simulink model "CVSG"  (R2024b)
settings: Solver=ode4  StartTime=0.0  StopTime=60  FixedStep=1e-5  RelTol=1e-3
values from neighbouring files (symbols this model uses):
  Dp = 2.087054162363824e+03    (= 2087.05416236)    [CVSGm.m]
  Dq = 0.686969675951841    (= 0.686969675952)    [CVSGm.m]
  Kp = 0.007666307989764    (= 0.00766630798976)    [CVSGm.m]
  Kq = 0.115300461672244    (= 0.115300461672)    [CVSGm.m]
undefined symbols (not defined in the file or in its folder): Filter, Ls, params
libraries: spsCurrentMeasurementLib x6, spsParallelRLCBranchLib x6, spsIGBTDiodeLib x6, spsSeriesRLCBranchLib x6, simulink x4, spsVoltageMeasurementLib x4, spsVariableInductorLib x3, spsVariableResistorLib x3, spsMeanLib x2, spsDCVoltageSourceLib x1, spsThreePhaseSourceLib x1, spsThreePhaseVIMeasurementLib x1
settings Model: SimulationMode=accelerator  Creator=Admin  LastModifiedBy=ACER
settings DataIOCC: SaveOutput=off  DSMLogging=off  SaveTime=off  ReturnWorkspaceOutputs=off
settings OptimizationCC: EfficientMapNaN2IntZero=off  AccelVerboseBuild=on
settings DebuggingCC: SignalInfNanChecking=error  CheckMatrixSingularityMsg=error  UnconnectedInputMsg=warning  UnconnectedOutputMsg=warning  UnconnectedLineMsg=warning
settings HardwareCC: TargetBitPerPointer=64  TargetBitPerSizeT=64  TargetBitPerPtrDiffT=64  TargetLongLongMode=on  TargetIntDivRoundTo=Zero  TargetEndianess=LittleEndian  TargetWordSize=64  TargetHWDeviceType=MATLAB Host  ProdEqTarget=off
settings ModelReferenceCC: EnableRefExpFcnMdlSchedulingChecks=on
settings SFSimCC: CustomCodeUndefinedFunction=UseInterfaceOnly
settings RTWCC: GPUComputeCapability=3.5
settings CodeAppCC: MaxIdLength=128
settings GRTTargetCC: TargetLangStandard=C89/C90 (ANSI)  CombineOutputUpdateFcns=off  GRTInterface=on

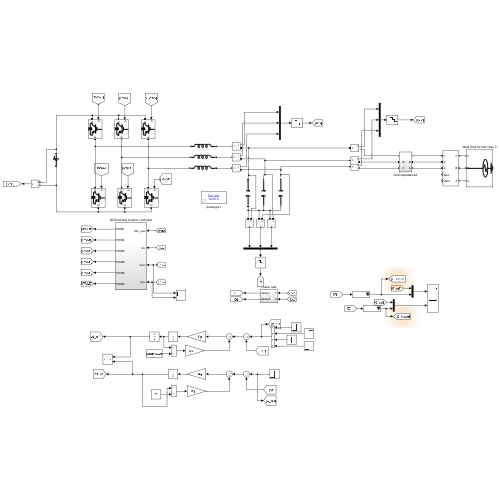
[thumbnail: Simulink's stored preview of the top-level diagram]
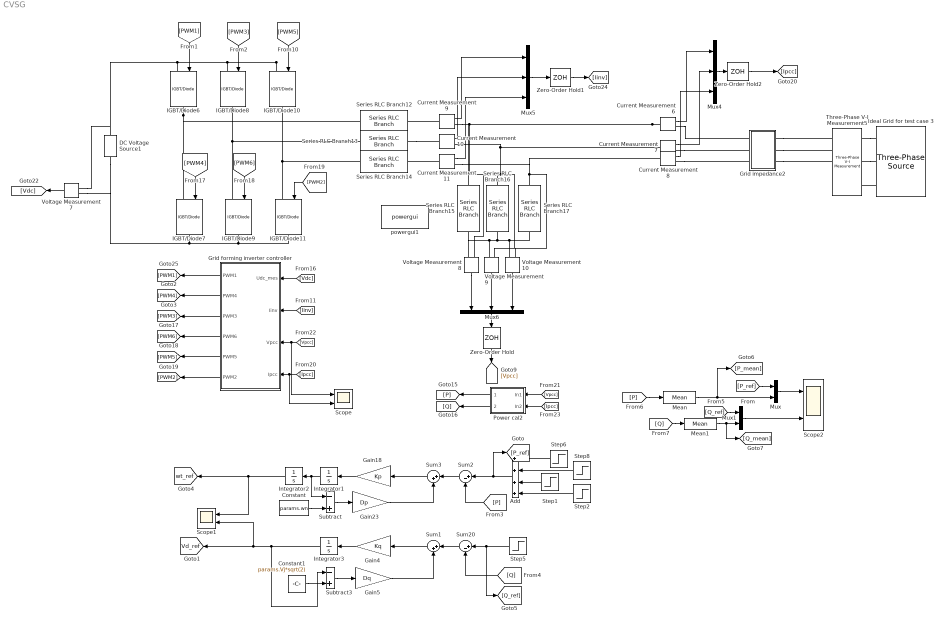
== system CVSG ==
  Add : Sum  Inputs=++++
  Constant : Constant  Value=params.wn
  Constant1 : Constant  Value=params.Vj*sqrt(2)
  Current Measurement{6..11} (6 alike) : spsCurrentMeasurementLib/Current Measurement  PhasorSimulation=off  OutputType=Complex  PSBequivalent=0
  DC Voltage Source1 : spsDCVoltageSourceLib/DC Voltage Source  Amplitude=params.Vdc  Measurements=None
  Gain18 : Gain  Gain=Kp
  Gain23 : Gain  Gain=Dp
  Gain4 : Gain  Gain=Kq
  Gain5 : Gain  Gain=Dq
  Grid forming inverter controller : Subsystem
  Grid impedance2 : Subsystem
  IGBT/Diode{6..11} (6 alike) : spsIGBTDiodeLib/IGBT//Diode  Ron=1e-3  Rs=1e5  Cs=inf  Measurements=off
  Ideal Grid for test case 3 : spsThreePhaseSourceLib/Three-Phase Source  InternalConnection=Yg  VoltagePhases=off  Voltage=params.Vj*sqrt(3)  PhaseAngle=0  Voltage_phases=[25e3 25e3 25e3]/sqrt(3)  PhaseAngles_phases=[0 -120 +120]  Frequency=params.f0  NonIdealSource=off  SpecifyImpedance=on  Resistance=0.8929  Inductance=16.58e-3  ShortCircuitLevel=params.SCR*params.S_rated  BaseVoltage=params.Vll_rms  XRratio=params.XR  BusType=swing  Pref=1e3  Qref=0  Prefabc=[10e3, 10e3, 10e3]  Qrefabc=[0, 0, 0]  Qmin=-inf  Qmax=inf
  Integrator1 : Integrator
  Integrator2 : Integrator
  Integrator3 : Integrator
  Mean : spsMeanLib/Mean  Freq=60  Vinit=0  Ts=0
  Mean1 : spsMeanLib/Mean  Freq=60  Vinit=0  Ts=0
  Mux : Mux  Inputs=2
  Mux1 : Mux  Inputs=2
  Mux4 : Mux  Inputs=3
  Mux5 : Mux  Inputs=3
  Mux6 : Mux  Inputs=3
  Power cal2 : Subsystem
  Scope : Scope  NumInputPorts=2
  Scope1 : Scope  NumInputPorts=2
  Scope2 : Scope  NumInputPorts=2
  Series RLC Branch12 : spsSeriesRLCBranchLib/Series RLC Branch  LConnTagsString=__new0  RConnTagsString=__new0  BranchType=L  Resistance=Filter.Rs_1  Inductance=params.Filter.Ls_1  SetiL0=off  InitialCurrent=1  Capacitance=1e-6  Setx0=off  InitialVoltage=0  Measurements=None
  Series RLC Branch13 : spsSeriesRLCBranchLib/Series RLC Branch  LConnTagsString=__new0  RConnTagsString=__new0  BranchType=L  Resistance=Filter.Rs_1  Inductance=params.Filter.Ls_1  SetiL0=off  InitialCurrent=1  Capacitance=1e-6  Setx0=off  InitialVoltage=0  Measurements=None
  Series RLC Branch14 : spsSeriesRLCBranchLib/Series RLC Branch  LConnTagsString=__new0  RConnTagsString=__new0  BranchType=L  Resistance=Filter.Rs_1  Inductance=params.Filter.Ls_1  SetiL0=off  InitialCurrent=1  Capacitance=1e-6  Setx0=off  InitialVoltage=0  Measurements=None
  Series RLC Branch15 : spsSeriesRLCBranchLib/Series RLC Branch  LConnTagsString=__new0  RConnTagsString=__new0  BranchType=C  Resistance=1  Inductance=Ls  SetiL0=off  InitialCurrent=0  Capacitance=params.Filter.Cs  Setx0=off  InitialVoltage=0  Measurements=None
  Series RLC Branch16 : spsSeriesRLCBranchLib/Series RLC Branch  LConnTagsString=__new0  RConnTagsString=__new0  BranchType=C  Resistance=1  Inductance=Ls  SetiL0=off  InitialCurrent=0  Capacitance=params.Filter.Cs  Setx0=off  InitialVoltage=0  Measurements=None
  Series RLC Branch17 : spsSeriesRLCBranchLib/Series RLC Branch  LConnTagsString=__new0  RConnTagsString=__new0  BranchType=C  Resistance=1  Inductance=Ls  SetiL0=off  InitialCurrent=0  Capacitance=params.Filter.Cs  Setx0=off  InitialVoltage=0  Measurements=None
  Step1 : Step  Time=70  After=0.5e3  SampleTime=0
  Step2 : Step  Time=70  After=0.5e3  SampleTime=0
  Step5 : Step  Time=50  Before=1e3  After=1.5e3  SampleTime=0
  Step6 : Step  Time=10  Before=2e3  After=2.5e3  SampleTime=0
  Step8 : Step  Time=30  After=0.5e3  SampleTime=0
  Subtract : Sum  Inputs=-+
  Subtract3 : Sum  Inputs=-+
  Sum1 : Sum  Inputs=|++
  Sum2 : Sum  Inputs=|+-
  Sum20 : Sum  Inputs=|+-
  Sum3 : Sum  Inputs=|++
  Three-Phase V-I Measurement5 : spsThreePhaseVIMeasurementLib/Three-Phase V-I Measurement  VoltageMeasurement=phase-to-ground  SetLabelV=off  LabelV=Vabc  Vpu=off  VpuLL=off  CurrentMeasurement=yes  SetLabelI=off  LabelI=Iabc  Ipu=off  Pbase=100e6  Vbase=500e3  OutputType=Complex  PhasorSimulation=off  PSBequivalent=0
  Voltage Measurement{7..10} (4 alike) : spsVoltageMeasurementLib/Voltage Measurement  PhasorSimulation=off  OutputType=Complex  PSBequivalent=0
  Zero-Order Hold : ZeroOrderHold  SampleTime=5e-5
  Zero-Order Hold1 : ZeroOrderHold  SampleTime=5e-5
  Zero-Order Hold2 : ZeroOrderHold  SampleTime=5e-5
  powergui1 : sps_lib/powergui  Priority=1  SimulationMode=Discrete  SampleTime=1e-5  frequency=60  Iterations=50  frequencyindice=0  Pbase=100e6  ErrMax=1e-4  UnitsV=kV  UnitsW=MW  buscounter=0  FunctionMessages=off  echomessages=off  EnableUseOfTLC=off  CurrentSourceSwitches=off  DisableSnubberDevices=off  DisableRonSwitches=off  DisableVfSwitches=off  DisplayEquations=off  AutomaticDiscreteSolvers=on  SolverType=Tustin/Backward Euler (TBE)  Interpol=off  ExternalGateDelay=off  methode=off  Ts=100  x0status=blocks  SPID=on  SwTol=0  HookPort=off  NonlinearTolerance=0  nMaxIteration=15  ContinueOnMaxIteration=off  RestoreLinks=warning  ResistiveCurrentMeasurement=off  Frange=[0:2:500]  Ylog=off  Xlog=on  ShowGrid=off  save=off  variable=ZData  structure=0  ZoomFFT=off  StartTime=0.0  cycles=1  DisplayStyle=1  fundamental=60  FreqAxis=off  MaxFrequency=1000  frequencyindicesteady=1  RmsSteady=1  display=off
  tag scope: Vd_ref=global, wt_ref=global
  wires:
  [Iinv] -> Grid forming inverter controller/2(Iinv)
  Grid forming inverter controller/1(PWM1) -> [PWM1]
  Grid forming inverter controller/4("PWM6 ") -> [PWM6]
  Grid forming inverter controller/6(PWM2) -> [PWM2]
  Voltage Measurement7/1 -> [Vdc]
  Grid forming inverter controller/5(PWM5) -> [PWM5]
  Voltage Measurement9/1 -> Mux6/2
  Mux5/1 -> Zero-Order Hold1/1
  [PWM6] -> IGBT/Diode9/1
  [PWM1] -> IGBT/Diode6/1
  [Ipcc] -> Scope/2, Grid forming inverter controller/4(Ipcc)
  [Vdc] -> Grid forming inverter controller/1(Udc_mes)
  [Vpcc] -> Scope/1, Grid forming inverter controller/3(Vpcc)
  Grid forming inverter controller/3(PWM3) -> [PWM3]
  Grid forming inverter controller/2("PWM4 ") -> [PWM4]
  Current Measurement11/1 -> Mux5/3
  Voltage Measurement10/1 -> Mux6/3
  [PWM2] -> IGBT/Diode11/1
  Mux4/1 -> Zero-Order Hold2/1
  [PWM4] -> IGBT/Diode7/1
  Mux6/1 -> Zero-Order Hold/1
  [PWM5] -> IGBT/Diode10/1
  Current Measurement8/1 -> Mux4/3
  Voltage Measurement8/1 -> Mux6/1
  Current Measurement9/1 -> Mux5/1
  Current Measurement7/1 -> Mux4/2
  Current Measurement6/1 -> Mux4/1
  Current Measurement10/1 -> Mux5/2
  [PWM3] -> IGBT/Diode8/1
  Power cal2/2(deltay2) -> [Q]
  Power cal2/1(deltay1) -> [P]
  [Vpcc] -> Power cal2/1(In1)
  [Ipcc] -> Power cal2/2(In2)
  Zero-Order Hold/1 -> [Vpcc]
  Zero-Order Hold1/1 -> [Iinv]
  Zero-Order Hold2/1 -> [Ipcc]
  Step8/1 -> Add/2
  Constant/1 -> Subtract/2
  Gain18/1 -> Integrator1/1
  Sum1/1 -> Gain4/1
  Gain5/1 -> Sum1/2
  Sum3/1 -> Gain18/1
  [Q] -> Sum20/2
  Integrator1/1 -> Subtract/1, Integrator2/1
  Constant1/1 -> Subtract3/2
  [P] -> Sum2/2
  Sum2/1 -> Sum3/1
  Integrator3/1 -> Scope1/2, [Vd_ref], Subtract3/1
  Sum20/1 -> Sum1/1
  Integrator2/1 -> [wt_ref], Scope1/1
  Subtract/1 -> Gain23/1
  Gain4/1 -> Integrator3/1
  Gain23/1 -> Sum3/2
  Subtract3/1 -> Gain5/1
  Mux/1 -> Scope2/1
  Mux1/1 -> Scope2/2
  Mean/1 -> [P_mean], Mux/2
  [P_ref] -> Mux/1
  [Q_ref] -> Mux1/1
  [P] -> Mean/1
  [Q] -> Mean1/1
  Step6/1 -> Add/1
  Add/1 -> [P_ref], Sum2/1
  Step1/1 -> Add/3
  Step2/1 -> Add/4
  Step5/1 -> [Q_ref], Sum20/1
  Mean1/1 -> [Q_mean], Mux1/2
  connections:
  Series RLC Branch14/LConn1 -- IGBT/Diode10/RConn1 -- IGBT/Diode11/LConn1
  Series RLC Branch17/LConn1 -- Current Measurement11/RConn1 -- Current Measurement8/LConn1 -- Voltage Measurement10/LConn1
  IGBT/Diode6/RConn1 -- Series RLC Branch12/LConn1 -- IGBT/Diode7/LConn1
  Voltage Measurement10/LConn2 -- Series RLC Branch17/RConn1 -- Voltage Measurement8/LConn2 -- Series RLC Branch15/RConn1 -- Voltage Measurement9/LConn2 -- Series RLC Branch16/RConn1
  Current Measurement6/LConn1 -- Series RLC Branch15/LConn1 -- Voltage Measurement8/LConn1 -- Current Measurement9/RConn1
  IGBT/Diode10/LConn1 -- DC Voltage Source1/RConn1 -- Voltage Measurement7/LConn1 -- IGBT/Diode6/LConn1 -- IGBT/Diode8/LConn1
  IGBT/Diode7/RConn1 -- IGBT/Diode11/RConn1 -- IGBT/Diode9/RConn1 -- Voltage Measurement7/LConn2 -- DC Voltage Source1/LConn1
  Series RLC Branch13/LConn1 -- IGBT/Diode8/RConn1 -- IGBT/Diode9/LConn1
  Current Measurement7/LConn1 -- Current Measurement10/RConn1 -- Series RLC Branch16/LConn1 -- Voltage Measurement9/LConn1
  Current Measurement7/RConn1 -- Grid impedance2/LConn2
  Current Measurement11/LConn1 -- Series RLC Branch14/RConn1
  Current Measurement8/RConn1 -- Grid impedance2/LConn3
  Series RLC Branch13/RConn1 -- Current Measurement10/LConn1
  Current Measurement9/LConn1 -- Series RLC Branch12/RConn1
  Current Measurement6/RConn1 -- Grid impedance2/LConn1
  Grid impedance2/RConn1 -- Three-Phase V-I Measurement5/RConn3
  Three-Phase V-I Measurement5/LConn2 -- Ideal Grid for test case 3/RConn2
  Three-Phase V-I Measurement5/LConn3 -- Ideal Grid for test case 3/RConn3
  Grid impedance2/RConn2 -- Three-Phase V-I Measurement5/RConn2
  Ideal Grid for test case 3/RConn1 -- Three-Phase V-I Measurement5/LConn1
  Grid impedance2/RConn3 -- Three-Phase V-I Measurement5/RConn1

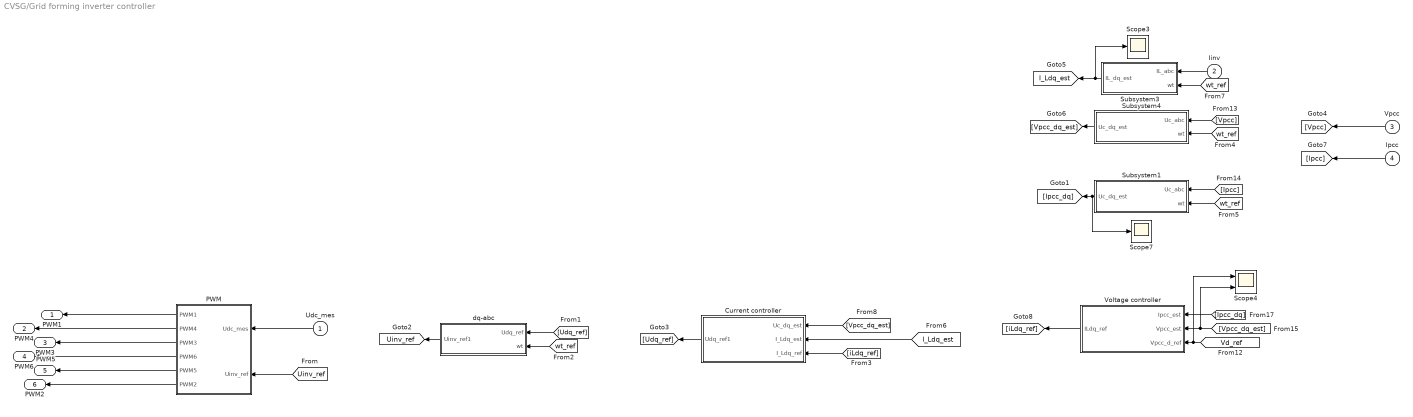
== system CVSG/Grid forming inverter controller ==
  Udc_mes : Inport
  Iinv : Inport  Port=2
  Vpcc : Inport  Port=3
  Ipcc : Inport  Port=4
  Current controller : Subsystem
  PWM : Subsystem
  Scope3 : Scope
  Scope4 : Scope  NumInputPorts=2
  Scope7 : Scope
  Subsystem1 : Subsystem
  Subsystem3 : Subsystem
  Subsystem4 : Subsystem
  Voltage controller : Subsystem
  dq-abc : Subsystem
  PWM1 : Outport
  "PWM4 " : Outport  Port=2
  PWM3 : Outport  Port=3
  "PWM6 " : Outport  Port=4
  PWM5 : Outport  Port=5
  PWM2 : Outport  Port=6
  tag scope: I_Ldq_est=global, Uinv_ref=global
  wires:
  [Vpcc_dq_est] -> Current controller/1(Uc_dq_est)
  PWM/4("PWM6 ") -> "PWM6 "/1
  Udc_mes/1 -> PWM/1(Udc_mes)
  [I_Ldq_est] -> Current controller/2(I_Ldq_est)
  Subsystem4/1(Uc_dq_est) -> [Vpcc_dq_est]
  Current controller/1(Udq_ref1) -> [Udq_ref]
  [wt_ref] -> Subsystem3/2(wt)
  dq-abc/1(Uinv_ref1) -> [Uinv_ref]
  [wt_ref] -> dq-abc/2(wt)
  Iinv/1 -> Subsystem3/1(IL_abc)
  PWM/3(PWM3) -> PWM3/1
  Subsystem3/1(IL_dq_est) -> Scope3/1, [I_Ldq_est]
  [wt_ref] -> Subsystem4/2(wt)
  PWM/1(PWM1) -> PWM1/1
  PWM/5(PWM5) -> PWM5/1
  PWM/6(PWM2) -> PWM2/1
  PWM/2("PWM4 ") -> "PWM4 "/1
  [Udq_ref] -> dq-abc/1(Udq_ref)
  [Uinv_ref] -> PWM/2(Uinv_ref)
  [Ipcc_dq] -> Voltage controller/1(Ipcc_est)
  Voltage controller/1(ILdq_ref) -> [iLdq_ref]
  [Vpcc_dq_est] -> Scope4/2, Voltage controller/2(Vpcc_est)
  [iLdq_ref] -> Current controller/3(I_Ldq_ref)
  [wt_ref] -> Subsystem1/2(wt)
  Subsystem1/1(Uc_dq_est) -> [Ipcc_dq], Scope7/1
  Vpcc/1 -> [Vpcc]
  Ipcc/1 -> [Ipcc]
  [Vpcc] -> Subsystem4/1(Uc_abc)
  [Ipcc] -> Subsystem1/1(Uc_abc)
  [Vd_ref] -> Scope4/1, Voltage controller/3(Vpcc_d_ref)

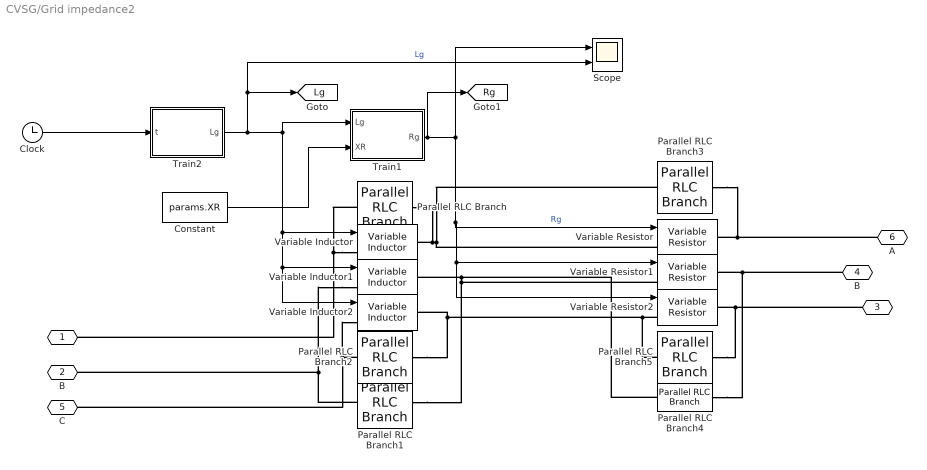
== system CVSG/Grid impedance2 ==
  Clock : Clock
      settings: Decimation=150
  Constant : Constant  Value=params.XR
  Parallel RLC Branch{,1..5} (6 alike) : spsParallelRLCBranchLib/Parallel RLC Branch  LConnTagsString=a  RConnTagsString=__new0  BranchType=R  Resistance=1e6  Inductance=1e-3  SetiL0=off  InitialCurrent=0  Capacitance=1e-6  Setx0=off  InitialVoltage=0  Measurements=None
  Scope : Scope  NumInputPorts=2
  Train1 : MATLAB Function  TreatAsAtomicUnit=on
  Train2 : MATLAB Function  TreatAsAtomicUnit=on
  Variable Inductor : spsVariableInductorLib/Variable Inductor  methode=Backward Euler  Labsmin=1e-6  Initialize=off  iL0=0  L0=1e-3  Vl0=-0.0024759
  Variable Inductor1 : spsVariableInductorLib/Variable Inductor  methode=Backward Euler  Labsmin=1e-6  Initialize=off  iL0=0  L0=1e-3  Vl0=67.3622
  Variable Inductor2 : spsVariableInductorLib/Variable Inductor  methode=Backward Euler  Labsmin=1e-6  Initialize=off  iL0=0  L0=1e-3  Vl0=-67.3597
  Variable Resistor : spsVariableResistorLib/Variable Resistor  Rabsmin=1e-3
  Variable Resistor1 : spsVariableResistorLib/Variable Resistor  Rabsmin=1e-3
  Variable Resistor2 : spsVariableResistorLib/Variable Resistor  Rabsmin=1e-3
  "   " : PMIOPort  Side=Left
  "   B" : PMIOPort  Port=2  Side=Left
  "  " : PMIOPort  Port=3  Side=Right
  "  B" : PMIOPort  Port=4  Side=Right
  "   C" : PMIOPort  Port=5  Side=Left
  "  A" : PMIOPort  Port=6  Side=Right
  tag scope: Lg=global, Rg=global
  wires:
  Train1/1(Rg) -> [Rg], Scope/1, Variable Resistor/1, Variable Resistor1/1, Variable Resistor2/1  "Rg"
  Clock/1 -> Train2/1(t)
  Train2/1(Lg) -> [Lg], Scope/2, Variable Inductor/1, Variable Inductor1/1, Variable Inductor2/1, Train1/1(Lg)  "Lg"
  Constant/1 -> Train1/2(XR)
  connections:
  Variable Resistor1/LConn1 -- Variable Inductor1/RConn1 -- Parallel RLC Branch4/LConn1 -- Parallel RLC Branch1/RConn1
  Variable Resistor2/LConn1 -- Parallel RLC Branch5/LConn1 -- Variable Inductor2/RConn1 -- Parallel RLC Branch2/RConn1
  Variable Resistor1/RConn1 -- Parallel RLC Branch4/RConn1 -- "  B"/RConn1
  Variable Resistor2/RConn1 -- Parallel RLC Branch5/RConn1 -- "  "/RConn1
  Variable Resistor/RConn1 -- Parallel RLC Branch3/RConn1 -- "  A"/RConn1
  Variable Inductor/LConn1 -- "   "/RConn1 -- Parallel RLC Branch/LConn1
  Variable Inductor/RConn1 -- Parallel RLC Branch3/LConn1 -- Variable Resistor/LConn1 -- Parallel RLC Branch/RConn1
  Variable Inductor1/LConn1 -- "   B"/RConn1 -- Parallel RLC Branch1/LConn1
  Variable Inductor2/LConn1 -- "   C"/RConn1 -- Parallel RLC Branch2/LConn1

== system CVSG/Power cal2 ==
  In1 : Inport
  In2 : Inport  Port=2
  Demux10 : Demux  Outputs=3
  Demux11 : Demux  Outputs=3
  Subsystem8 : Subsystem
  Subsystem9 : Subsystem
  p3 : Subsystem
  q3 : Subsystem
  deltay1 : Outport
  deltay2 : Outport  Port=2
  wires:
  In1/1 -> Demux11/1
  In2/1 -> Demux10/1
  q3/1(deltay2) -> deltay2/1
  Demux10/1 -> Subsystem8/1(xa)
  Demux11/2 -> Subsystem9/2(xb)
  Demux11/1 -> Subsystem9/1(xa)
  Subsystem9/2(xbeta) -> q3/2(Beta), p3/2(Beta)
  p3/1(deltay1) -> deltay1/1
  Demux10/3 -> Subsystem8/3(xc)
  Subsystem9/1(xalpha) -> q3/1(Alpha), p3/1(Alpha)
  Demux10/2 -> Subsystem8/2(xb)
  Subsystem8/2(xbeta) -> q3/4(xbeta), p3/4(xbeta)
  Demux11/3 -> Subsystem9/3(xc)
  Subsystem8/1(xalpha) -> q3/3(xalpha), p3/3(xalpha)

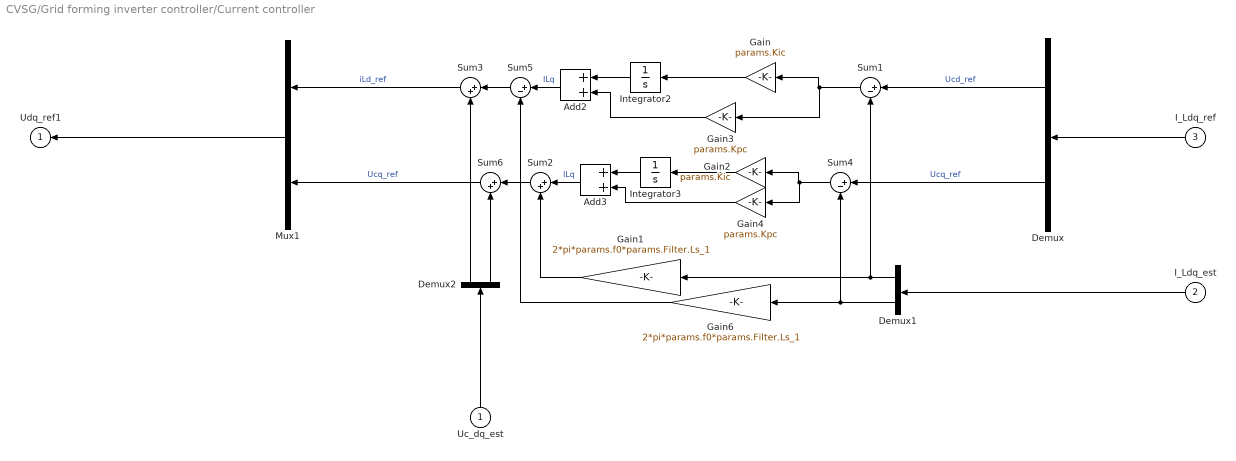
== system CVSG/Grid forming inverter controller/Current controller ==
  Uc_dq_est : Inport
  I_Ldq_est : Inport  Port=2
  I_Ldq_ref : Inport  Port=3
  Add2 : Sum
  Add3 : Sum
  Demux : Demux  Outputs=2
  Demux1 : Demux  Outputs=2
  Demux2 : Demux  Outputs=2
  Gain : Gain  Gain=params.Kic
  Gain1 : Gain  Gain=2*pi*params.f0*params.Filter.Ls_1
  Gain2 : Gain  Gain=params.Kic
  Gain3 : Gain  Gain=params.Kpc
  Gain4 : Gain  Gain=params.Kpc
  Gain6 : Gain  Gain=2*pi*params.f0*params.Filter.Ls_1
  Integrator2 : Integrator
  Integrator3 : Integrator
  Mux1 : Mux  Inputs=2
  Sum1 : Sum  Inputs=|+-
  Sum2 : Sum  Inputs=|++
  Sum3 : Sum  Inputs=|++
  Sum4 : Sum  Inputs=|+-
  Sum5 : Sum  Inputs=|+-
  Sum6 : Sum  Inputs=|++
  Udq_ref1 : Outport  InitialOutput=0  VectorParamsAs1DForOutWhenUnconnected=off
  wires:
  I_Ldq_ref/1 -> Demux/1
  Demux2/2 -> Sum6/2
  Sum2/1 -> Sum6/1
  I_Ldq_est/1 -> Demux1/1
  Sum3/1 -> Mux1/1  "iLd_ref"
  Demux/2 -> Sum4/1  "Ucq_ref"
  Gain1/1 -> Sum2/2
  Sum6/1 -> Mux1/2  "Ucq_ref"
  Demux2/1 -> Sum3/2
  Sum5/1 -> Sum3/1
  Mux1/1 -> Udq_ref1/1
  Gain6/1 -> Sum5/2
  Uc_dq_est/1 -> Demux2/1
  Demux1/2 -> Gain6/1, Sum4/2
  Demux/1 -> Sum1/1  "Ucd_ref"
  Demux1/1 -> Sum1/2, Gain1/1
  Add2/1 -> Sum5/1  "ILq"
  Add3/1 -> Sum2/1  "ILq"
  Integrator2/1 -> Add2/1
  Integrator3/1 -> Add3/1
  Gain/1 -> Integrator2/1
  Sum1/1 -> Gain3/1, Gain/1
  Gain2/1 -> Integrator3/1
  Sum4/1 -> Gain4/1, Gain2/1
  Gain3/1 -> Add2/2
  Gain4/1 -> Add3/2

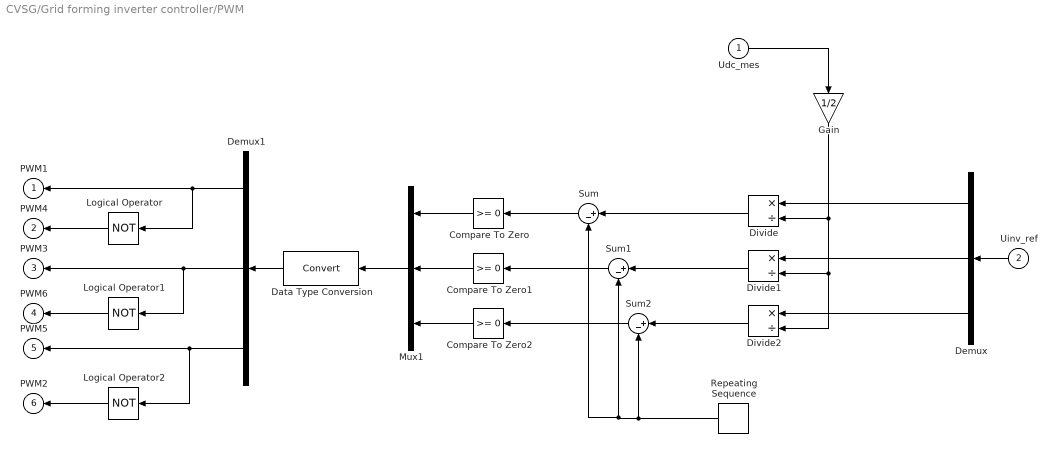
== system CVSG/Grid forming inverter controller/PWM ==
  Udc_mes : Inport
  Uinv_ref : Inport  Port=2
  Compare To Zero : simulink/Logic and Bit Operations/Compare To Zero  relop=>=  OutDataTypeStr=boolean
  Compare To Zero1 : simulink/Logic and Bit Operations/Compare To Zero  relop=>=  OutDataTypeStr=boolean
  Compare To Zero2 : simulink/Logic and Bit Operations/Compare To Zero  relop=>=  OutDataTypeStr=boolean
  Data Type Conversion : DataTypeConversion  SaturateOnIntegerOverflow=off  RndMeth=Floor
  Demux : Demux  Outputs=3
  Demux1 : Demux  Outputs=3
  Divide : Product  Inputs=*/
  Divide1 : Product  Inputs=*/
  Divide2 : Product  Inputs=*/
  Gain : Gain  Gain=1/2
  Logical Operator : Logic  Operator=NOT  AllPortsSameDT=off  OutDataTypeStr=boolean
  Logical Operator1 : Logic  Operator=NOT  AllPortsSameDT=off  OutDataTypeStr=boolean
  Logical Operator2 : Logic  Operator=NOT  AllPortsSameDT=off  OutDataTypeStr=boolean
  Mux1 : Mux  Inputs=3
  Repeating Sequence : simulink/Sources/Repeating Sequence  rep_seq_t=[0 params.Ts/2 params.Ts]  rep_seq_y=[-1 1 -1]
  Sum : Sum  Inputs=|+-
  Sum1 : Sum  Inputs=|+-
  Sum2 : Sum  Inputs=|+-
  PWM1 : Outport  InitialOutput=0  VectorParamsAs1DForOutWhenUnconnected=off
  "PWM4 " : Outport  Port=2  InitialOutput=0  VectorParamsAs1DForOutWhenUnconnected=off
  PWM3 : Outport  Port=3  InitialOutput=0  VectorParamsAs1DForOutWhenUnconnected=off
  "PWM6 " : Outport  Port=4  InitialOutput=0  VectorParamsAs1DForOutWhenUnconnected=off
  PWM5 : Outport  Port=5  InitialOutput=0  VectorParamsAs1DForOutWhenUnconnected=off
  PWM2 : Outport  Port=6  InitialOutput=0  VectorParamsAs1DForOutWhenUnconnected=off
  wires:
  Repeating Sequence/1 -> Sum/2, Sum1/2, Sum2/2
  Sum1/1 -> Compare To Zero1/1
  Mux1/1 -> Data Type Conversion/1
  Divide2/1 -> Sum2/1
  Divide/1 -> Sum/1
  Logical Operator/1 -> "PWM4 "/1
  Sum2/1 -> Compare To Zero2/1
  Divide1/1 -> Sum1/1
  Demux/1 -> Divide/1
  Uinv_ref/1 -> Demux/1
  Demux1/2 -> PWM3/1, Logical Operator1/1
  Demux1/3 -> PWM5/1, Logical Operator2/1
  Compare To Zero2/1 -> Mux1/3
  Compare To Zero1/1 -> Mux1/2
  Demux/2 -> Divide1/1
  Logical Operator2/1 -> PWM2/1
  Logical Operator1/1 -> "PWM6 "/1
  Udc_mes/1 -> Gain/1
  Demux/3 -> Divide2/1
  Sum/1 -> Compare To Zero/1
  Gain/1 -> Divide/2, Divide1/2, Divide2/2
  Demux1/1 -> PWM1/1, Logical Operator/1
  Data Type Conversion/1 -> Demux1/1
  Compare To Zero/1 -> Mux1/1

== system CVSG/Grid forming inverter controller/Subsystem1 ==
  Uc_abc : Inport
  wt : Inport  Port=2
  Demux : Demux  Outputs=3
  Mux1 : Mux  Inputs=2
  Subsystem1 : Subsystem
  Subsystem2 : Subsystem
  Uc_dq_est : Outport  InitialOutput=0  VectorParamsAs1DForOutWhenUnconnected=off
  wires:
  Mux1/1 -> Uc_dq_est/1
  wt/1 -> Subsystem2/3(wt)
  Demux/3 -> Subsystem1/3(xc)
  Subsystem2/1(xd) -> Mux1/1
  Subsystem1/2(xbeta) -> Subsystem2/2(xbeta)
  Demux/1 -> Subsystem1/1(xa)
  Uc_abc/1 -> Demux/1
  Subsystem1/1(xalpha) -> Subsystem2/1(xalpha)
  Demux/2 -> Subsystem1/2(xb)
  Subsystem2/2(xq) -> Mux1/2

== system CVSG/Grid forming inverter controller/Subsystem3 ==
  IL_abc : Inport
  wt : Inport  Port=2
  Demux : Demux  Outputs=3
  Mux1 : Mux  Inputs=2
  Subsystem1 : Subsystem
  Subsystem2 : Subsystem
  IL_dq_est : Outport  InitialOutput=0  VectorParamsAs1DForOutWhenUnconnected=off
  wires:
  Demux/3 -> Subsystem1/3(xc)
  IL_abc/1 -> Demux/1
  wt/1 -> Subsystem2/3(wt)
  Demux/1 -> Subsystem1/1(xa)
  Subsystem1/2(xbeta) -> Subsystem2/2(xbeta)
  Mux1/1 -> IL_dq_est/1
  Demux/2 -> Subsystem1/2(xb)
  Subsystem1/1(xalpha) -> Subsystem2/1(xalpha)
  Subsystem2/2(xq) -> Mux1/2
  Subsystem2/1(xd) -> Mux1/1

== system CVSG/Grid forming inverter controller/Subsystem4 ==
  Uc_abc : Inport
  wt : Inport  Port=2
  Demux : Demux  Outputs=3
  Mux1 : Mux  Inputs=2
  Subsystem1 : Subsystem
  Subsystem2 : Subsystem
  Uc_dq_est : Outport  InitialOutput=0  VectorParamsAs1DForOutWhenUnconnected=off
  wires:
  Subsystem2/2(xq) -> Mux1/2
  Demux/2 -> Subsystem1/2(xb)
  Subsystem1/1(xalpha) -> Subsystem2/1(xalpha)
  Uc_abc/1 -> Demux/1
  Demux/1 -> Subsystem1/1(xa)
  Subsystem1/2(xbeta) -> Subsystem2/2(xbeta)
  Subsystem2/1(xd) -> Mux1/1
  Demux/3 -> Subsystem1/3(xc)
  wt/1 -> Subsystem2/3(wt)
  Mux1/1 -> Uc_dq_est/1

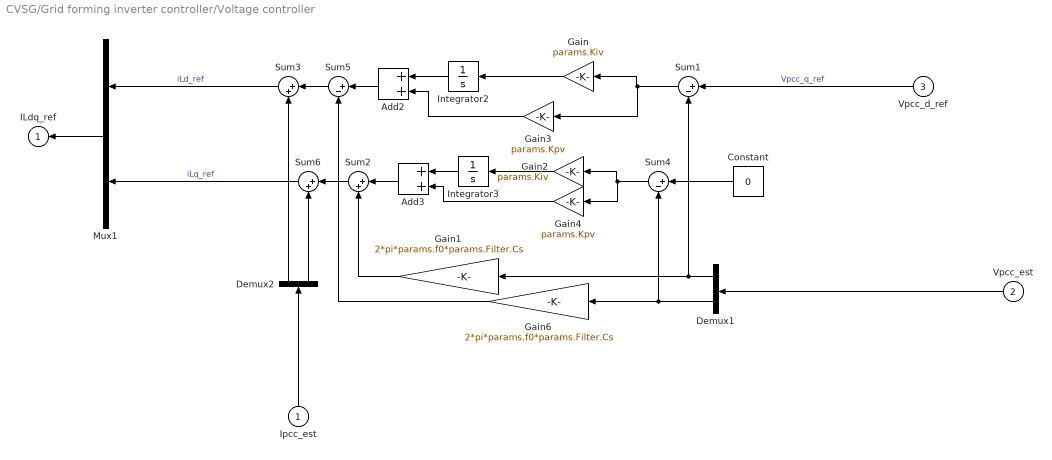
== system CVSG/Grid forming inverter controller/Voltage controller ==
  Ipcc_est : Inport
  Vpcc_est : Inport  Port=2
  Vpcc_d_ref : Inport  Port=3
  Add2 : Sum
  Add3 : Sum
  Constant : Constant  Value=0
  Demux1 : Demux  Outputs=2
  Demux2 : Demux  Outputs=2
  Gain : Gain  Gain=params.Kiv
  Gain1 : Gain  Gain=2*pi*params.f0*params.Filter.Cs
  Gain2 : Gain  Gain=params.Kiv
  Gain3 : Gain  Gain=params.Kpv
  Gain4 : Gain  Gain=params.Kpv
  Gain6 : Gain  Gain=2*pi*params.f0*params.Filter.Cs
  Integrator2 : Integrator
  Integrator3 : Integrator
  Mux1 : Mux  Inputs=2
  Sum1 : Sum  Inputs=|+-
  Sum2 : Sum  Inputs=|++
  Sum3 : Sum  Inputs=|++
  Sum4 : Sum  Inputs=|+-
  Sum5 : Sum  Inputs=|+-
  Sum6 : Sum  Inputs=|++
  ILdq_ref : Outport  InitialOutput=0  VectorParamsAs1DForOutWhenUnconnected=off
  wires:
  Gain4/1 -> Add3/2
  Gain3/1 -> Add2/2
  Sum4/1 -> Gain2/1, Gain4/1
  Gain2/1 -> Integrator3/1
  Sum1/1 -> Gain/1, Gain3/1
  Gain/1 -> Integrator2/1
  Integrator3/1 -> Add3/1
  Integrator2/1 -> Add2/1
  Add3/1 -> Sum2/1
  Add2/1 -> Sum5/1
  Demux1/1 -> Gain1/1, Sum1/2
  Demux1/2 -> Sum4/2, Gain6/1
  Ipcc_est/1 -> Demux2/1
  Gain6/1 -> Sum5/2
  Mux1/1 -> ILdq_ref/1
  Sum5/1 -> Sum3/1
  Demux2/1 -> Sum3/2
  Sum6/1 -> Mux1/2  "iLq_ref"
  Gain1/1 -> Sum2/2
  Sum3/1 -> Mux1/1  "iLd_ref"
  Vpcc_est/1 -> Demux1/1
  Sum2/1 -> Sum6/1
  Demux2/2 -> Sum6/2
  Vpcc_d_ref/1 -> Sum1/1  "Vpcc_q_ref"
  Constant/1 -> Sum4/1

== system CVSG/Grid forming inverter controller/dq-abc ==
  Udq_ref : Inport
  wt : Inport  Port=2
  Subsystem2 : Subsystem
  Subsystem3 : Subsystem
  Uinv_ref1 : Outport  InitialOutput=0  VectorParamsAs1DForOutWhenUnconnected=off
  wires:
  wt/1 -> Subsystem2/2(wt)
  Subsystem2/1(xalbe) -> Subsystem3/1(xalbe)
  Subsystem3/1(xabc) -> Uinv_ref1/1
  Udq_ref/1 -> Subsystem2/1(xdq)

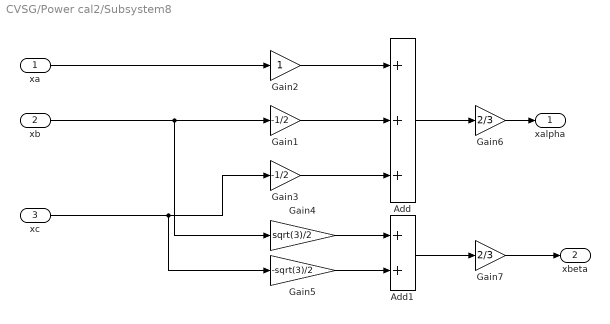
== system CVSG/Power cal2/Subsystem8 ==
  xa : Inport
  xb : Inport  Port=2
  xc : Inport  Port=3
  Add : Sum  Inputs=+++
  Add1 : Sum
  Gain1 : Gain  Gain=-1/2
  Gain2 : Gain
  Gain3 : Gain  Gain=-1/2
  Gain4 : Gain  Gain=sqrt(3)/2
  Gain5 : Gain  Gain=-sqrt(3)/2
  Gain6 : Gain  Gain=2/3
  Gain7 : Gain  Gain=2/3
  xalpha : Outport  VectorParamsAs1DForOutWhenUnconnected=off
  xbeta : Outport  Port=2  VectorParamsAs1DForOutWhenUnconnected=off
  wires:
  xc/1 -> Gain5/1, Gain3/1
  Gain6/1 -> xalpha/1
  Add1/1 -> Gain7/1
  Gain3/1 -> Add/3
  Gain1/1 -> Add/2
  xb/1 -> Gain4/1, Gain1/1
  Gain5/1 -> Add1/2
  Gain2/1 -> Add/1
  Add/1 -> Gain6/1
  Gain4/1 -> Add1/1
  Gain7/1 -> xbeta/1
  xa/1 -> Gain2/1

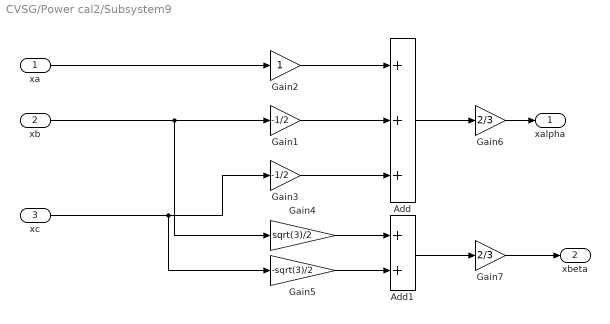
== system CVSG/Power cal2/Subsystem9 ==
  xa : Inport
  xb : Inport  Port=2
  xc : Inport  Port=3
  Add : Sum  Inputs=+++
  Add1 : Sum
  Gain1 : Gain  Gain=-1/2
  Gain2 : Gain
  Gain3 : Gain  Gain=-1/2
  Gain4 : Gain  Gain=sqrt(3)/2
  Gain5 : Gain  Gain=-sqrt(3)/2
  Gain6 : Gain  Gain=2/3
  Gain7 : Gain  Gain=2/3
  xalpha : Outport  VectorParamsAs1DForOutWhenUnconnected=off
  xbeta : Outport  Port=2  VectorParamsAs1DForOutWhenUnconnected=off
  wires:
  xa/1 -> Gain2/1
  Gain7/1 -> xbeta/1
  Gain4/1 -> Add1/1
  Add/1 -> Gain6/1
  Gain2/1 -> Add/1
  Gain5/1 -> Add1/2
  xb/1 -> Gain1/1, Gain4/1
  Gain1/1 -> Add/2
  Gain3/1 -> Add/3
  Add1/1 -> Gain7/1
  Gain6/1 -> xalpha/1
  xc/1 -> Gain3/1, Gain5/1

== system CVSG/Power cal2/p3 ==
  Alpha : Inport
  Beta : Inport  Port=2
  xalpha : Inport  Port=3
  xbeta : Inport  Port=4
  Add : Sum
  Gain : Gain  Gain=3/2
  Product : Product
  Product1 : Product
  deltay1 : Outport
  wires:
  Product1/1 -> Add/2
  Gain/1 -> deltay1/1
  Product/1 -> Add/1
  Add/1 -> Gain/1
  Alpha/1 -> Product/1
  xalpha/1 -> Product/2
  Beta/1 -> Product1/1
  xbeta/1 -> Product1/2

== system CVSG/Power cal2/q3 ==
  Alpha : Inport
  Beta : Inport  Port=2
  xalpha : Inport  Port=3
  xbeta : Inport  Port=4
  Add : Sum  Inputs=+-
  Gain : Gain  Gain=3/2
  Product : Product
  Product1 : Product
  deltay2 : Outport
  wires:
  Add/1 -> Gain/1
  Product/1 -> Add/1
  Gain/1 -> deltay2/1
  Product1/1 -> Add/2
  Beta/1 -> Product/1
  xalpha/1 -> Product/2
  Alpha/1 -> Product1/1
  xbeta/1 -> Product1/2

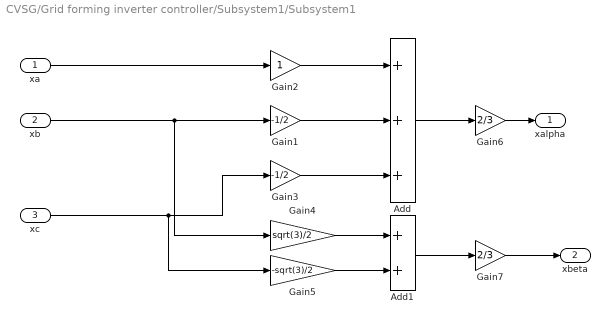
== system CVSG/Grid forming inverter controller/Subsystem1/Subsystem1 ==
  xa : Inport
  xb : Inport  Port=2
  xc : Inport  Port=3
  Add : Sum  Inputs=+++
  Add1 : Sum
  Gain1 : Gain  Gain=-1/2
  Gain2 : Gain
  Gain3 : Gain  Gain=-1/2
  Gain4 : Gain  Gain=sqrt(3)/2
  Gain5 : Gain  Gain=-sqrt(3)/2
  Gain6 : Gain  Gain=2/3
  Gain7 : Gain  Gain=2/3
  xalpha : Outport  VectorParamsAs1DForOutWhenUnconnected=off
  xbeta : Outport  Port=2  VectorParamsAs1DForOutWhenUnconnected=off
  wires:
  xa/1 -> Gain2/1
  Gain7/1 -> xbeta/1
  Gain4/1 -> Add1/1
  Add/1 -> Gain6/1
  Gain2/1 -> Add/1
  Gain5/1 -> Add1/2
  xb/1 -> Gain1/1, Gain4/1
  Gain1/1 -> Add/2
  Gain3/1 -> Add/3
  Add1/1 -> Gain7/1
  Gain6/1 -> xalpha/1
  xc/1 -> Gain3/1, Gain5/1

== system CVSG/Grid forming inverter controller/Subsystem1/Subsystem2 ==
  xalpha : Inport
  xbeta : Inport  Port=2
  wt : Inport  Port=3
  Fcn : Fcn  Expr=cos(u(3))*u(1)+u(2)*sin(u(3))
  Fcn1 : Fcn  Expr=-sin(u(3))*u(1)+u(2)*cos(u(3))
  Mux : Mux  Inputs=3
  xd : Outport  VectorParamsAs1DForOutWhenUnconnected=off
  xq : Outport  Port=2  VectorParamsAs1DForOutWhenUnconnected=off
  wires:
  wt/1 -> Mux/3
  xalpha/1 -> Mux/1
  Fcn1/1 -> xq/1
  xbeta/1 -> Mux/2
  Fcn/1 -> xd/1
  Mux/1 -> Fcn1/1, Fcn/1

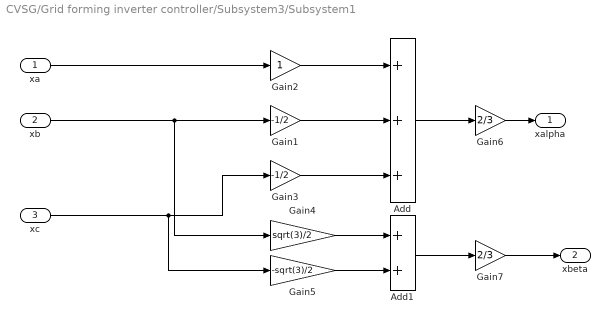
== system CVSG/Grid forming inverter controller/Subsystem3/Subsystem1 ==
  xa : Inport
  xb : Inport  Port=2
  xc : Inport  Port=3
  Add : Sum  Inputs=+++
  Add1 : Sum
  Gain1 : Gain  Gain=-1/2
  Gain2 : Gain
  Gain3 : Gain  Gain=-1/2
  Gain4 : Gain  Gain=sqrt(3)/2
  Gain5 : Gain  Gain=-sqrt(3)/2
  Gain6 : Gain  Gain=2/3
  Gain7 : Gain  Gain=2/3
  xalpha : Outport  VectorParamsAs1DForOutWhenUnconnected=off
  xbeta : Outport  Port=2  VectorParamsAs1DForOutWhenUnconnected=off
  wires:
  xc/1 -> Gain5/1, Gain3/1
  Gain6/1 -> xalpha/1
  Add1/1 -> Gain7/1
  Gain3/1 -> Add/3
  Gain1/1 -> Add/2
  xb/1 -> Gain4/1, Gain1/1
  Gain5/1 -> Add1/2
  Gain2/1 -> Add/1
  Add/1 -> Gain6/1
  Gain4/1 -> Add1/1
  Gain7/1 -> xbeta/1
  xa/1 -> Gain2/1

== system CVSG/Grid forming inverter controller/Subsystem3/Subsystem2 ==
  xalpha : Inport
  xbeta : Inport  Port=2
  wt : Inport  Port=3
  Fcn : Fcn  Expr=cos(u(3))*u(1)+u(2)*sin(u(3))
  Fcn1 : Fcn  Expr=-sin(u(3))*u(1)+u(2)*cos(u(3))
  Mux : Mux  Inputs=3
  xd : Outport  VectorParamsAs1DForOutWhenUnconnected=off
  xq : Outport  Port=2  VectorParamsAs1DForOutWhenUnconnected=off
  wires:
  wt/1 -> Mux/3
  Mux/1 -> Fcn/1, Fcn1/1
  Fcn/1 -> xd/1
  xbeta/1 -> Mux/2
  Fcn1/1 -> xq/1
  xalpha/1 -> Mux/1

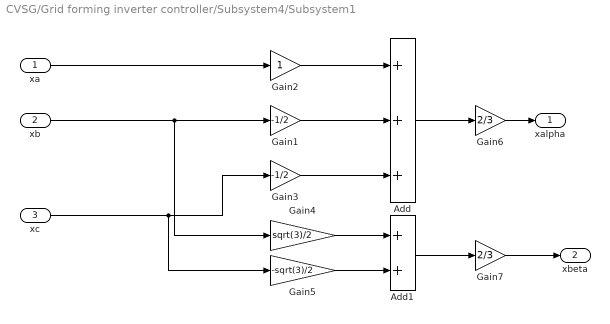
== system CVSG/Grid forming inverter controller/Subsystem4/Subsystem1 ==
  xa : Inport
  xb : Inport  Port=2
  xc : Inport  Port=3
  Add : Sum  Inputs=+++
  Add1 : Sum
  Gain1 : Gain  Gain=-1/2
  Gain2 : Gain
  Gain3 : Gain  Gain=-1/2
  Gain4 : Gain  Gain=sqrt(3)/2
  Gain5 : Gain  Gain=-sqrt(3)/2
  Gain6 : Gain  Gain=2/3
  Gain7 : Gain  Gain=2/3
  xalpha : Outport  VectorParamsAs1DForOutWhenUnconnected=off
  xbeta : Outport  Port=2  VectorParamsAs1DForOutWhenUnconnected=off
  wires:
  xc/1 -> Gain5/1, Gain3/1
  Gain6/1 -> xalpha/1
  Add1/1 -> Gain7/1
  Gain3/1 -> Add/3
  Gain1/1 -> Add/2
  xb/1 -> Gain4/1, Gain1/1
  Gain5/1 -> Add1/2
  Gain2/1 -> Add/1
  Add/1 -> Gain6/1
  Gain4/1 -> Add1/1
  Gain7/1 -> xbeta/1
  xa/1 -> Gain2/1

== system CVSG/Grid forming inverter controller/Subsystem4/Subsystem2 ==
  xalpha : Inport
  xbeta : Inport  Port=2
  wt : Inport  Port=3
  Fcn : Fcn  Expr=cos(u(3))*u(1)+u(2)*sin(u(3))
  Fcn1 : Fcn  Expr=-sin(u(3))*u(1)+u(2)*cos(u(3))
  Mux : Mux  Inputs=3
  xd : Outport  VectorParamsAs1DForOutWhenUnconnected=off
  xq : Outport  Port=2  VectorParamsAs1DForOutWhenUnconnected=off
  wires:
  Mux/1 -> Fcn/1, Fcn1/1
  Fcn/1 -> xd/1
  xbeta/1 -> Mux/2
  Fcn1/1 -> xq/1
  xalpha/1 -> Mux/1
  wt/1 -> Mux/3

== system CVSG/Grid forming inverter controller/dq-abc/Subsystem2 ==
  xdq : Inport
  wt : Inport  Port=2
  Demux : Demux  Outputs=2
  Fcn2 : Fcn  Expr=u(1)*cos(u(3))-u(2)*sin(u(3))
  Fcn3 : Fcn  Expr=u(1)*sin(u(3))+u(2)*cos(u(3))
  Mux : Mux  Inputs=2
  Mux2 : Mux  Inputs=3
  xalbe : Outport  VectorParamsAs1DForOutWhenUnconnected=off
  wires:
  Mux2/1 -> Fcn2/1, Fcn3/1
  wt/1 -> Mux2/3
  xdq/1 -> Demux/1
  Demux/1 -> Mux2/1
  Demux/2 -> Mux2/2
  Fcn2/1 -> Mux/1
  Fcn3/1 -> Mux/2
  Mux/1 -> xalbe/1

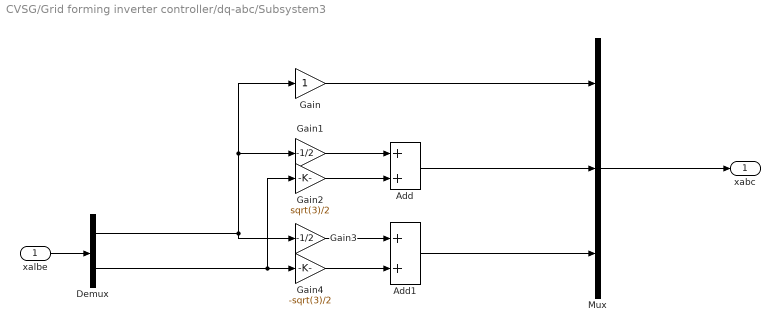
== system CVSG/Grid forming inverter controller/dq-abc/Subsystem3 ==
  xalbe : Inport
  Add : Sum
  Add1 : Sum
  Demux : Demux  Outputs=2
  Gain : Gain
  Gain1 : Gain  Gain=-1/2
  Gain2 : Gain  Gain=sqrt(3)/2
  Gain3 : Gain  Gain=-1/2
  Gain4 : Gain  Gain=-sqrt(3)/2
  Mux : Mux  Inputs=3
  xabc : Outport  VectorParamsAs1DForOutWhenUnconnected=off
  wires:
  Add1/1 -> Mux/3
  Demux/1 -> Gain/1, Gain1/1, Gain3/1
  Gain1/1 -> Add/1
  Add/1 -> Mux/2
  Demux/2 -> Gain2/1, Gain4/1
  Gain3/1 -> Add1/1
  Gain4/1 -> Add1/2
  Gain/1 -> Mux/1
  Gain2/1 -> Add/2
  Mux/1 -> xabc/1
  xalbe/1 -> Demux/1

== matlab function CVSG/Grid impedance2/Train1 ==
  data: Lg input; Rg output; XR input
function Rg = fcn(Lg, XR)
f0 = 50;
Rg = 2*pi*f0*Lg/XR;

== matlab function CVSG/Grid impedance2/Train2 ==
  data: t input; Lg output
function Lg = fcn(t)
    %— Tham số hệ thống ———————————————————————————————————
    Vll_rms = 110*sqrt(3);
    P_rated = 5000;
    w0       = 2*pi*50;

    %— Hồ sơ SCR & thời gian bước —————————————————————————
    persistent scr_vec step_T n_step
    if isempty(scr_vec)
        scr_vec = [2, 8, 20];
        step_T  = 20.0;            % mỗi bước 20 s
        n_step  = numel(scr_vec);
    end

    %— Chọn chỉ số bước bằng ceil ——————————————————————
    if t <= 0
        idx = 1;
    else
        idx = ceil(t / step_T);
        if idx > n_step
            idx = n_step;
        end
    end
    scr = scr_vec(idx);

    %— Tính Lg từ SCR —————————————————————————————
    Lg = Vll_rms^2 / ( scr * P_rated * w0 );
end
